simulink model "uc_faz_simetrik_PWM_simulink"  (R2019b)
settings: Solver=VariableStepAuto  StartTime=0.0  StopTime=0.02  RelTol=1e-3
values from neighbouring files (symbols this model uses):
  m = 0.70    (= 0.7)    [simetrikPWM_parametreleri.m]
  Ts = 1/2000    (= 0.0005)    [simetrikPWM_parametreleri.m]
  w = 2 * pi *50    (= 314.159265359)    [simetrikPWM_parametreleri.m]
libraries: powerlib x12
settings Model: Creator=Monster  LastModifiedBy=Monster

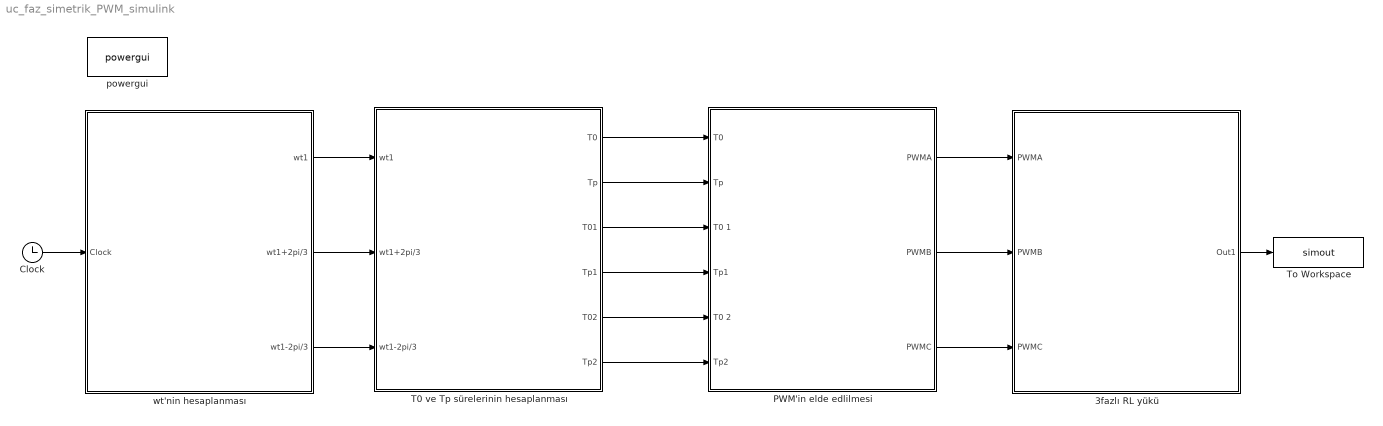
== system uc_faz_simetrik_PWM_simulink ==
  3fazlı RL yükü : Subsystem
  "Clock " : Clock
  PWM'in elde edlilmesi : Subsystem
  T0 ve Tp sürelerinin hesaplanması : Subsystem
  To Workspace : ToWorkspace  VariableName=simout  SaveFormat=Timeseries  SampleTime=-1
  "powergui " : powerlib/powergui  Priority=1  SimulationMode=Discrete  SampleTime=50e-6  frequency=60  Iterations=50  frequencyindice=0  Pbase=100e6  ErrMax=1e-4  UnitsV=kV  UnitsW=MW  buscounter=0  FunctionMessages=off  echomessages=off  EnableUseOfTLC=off  CurrentSourceSwitches=off  DisableSnubberDevices=off  DisableRonSwitches=off  DisableVfSwitches=off  DisplayEquations=off  AutomaticDiscreteSolvers=off  SolverType=Tustin/Backward Euler (TBE)  Interpol=off  ExternalGateDelay=off  methode=off  Ts=100  x0status=blocks  SPID=on  SwTol=0  HookPort=off  NonlinearTolerance=1e-4  nMaxIteration=100  ContinueOnMaxIteration=off  RestoreLinks=warning  ResistiveCurrentMeasurement=off  Frange=[0:2:500]  Ylog=off  Xlog=on  ShowGrid=off  save=off  variable=ZData  structure=0  ZoomFFT=off  StartTime=0.0  cycles=1  DisplayStyle=1  fundamental=60  FreqAxis=off  MaxFrequency=1000  frequencyindicesteady=1  RmsSteady=1  display=off
      settings: SourceProductName=Simscape Electrical
  wt'nin hesaplanması : Subsystem
  wires:
  "Clock "/1 -> wt'nin hesaplanması/1(Clock)
  wt'nin hesaplanması/1(wt1) -> T0 ve Tp sürelerinin hesaplanması/1(wt1)
  T0 ve Tp sürelerinin hesaplanması/1(T0) -> PWM'in elde edlilmesi/1("T0 ")
  T0 ve Tp sürelerinin hesaplanması/2(Tp) -> PWM'in elde edlilmesi/2(Tp)
  wt'nin hesaplanması/2(wt1+2pi/3) -> T0 ve Tp sürelerinin hesaplanması/2(wt1+2pi/3)
  wt'nin hesaplanması/3(wt1-2pi/3) -> T0 ve Tp sürelerinin hesaplanması/3(wt1-2pi/3)
  T0 ve Tp sürelerinin hesaplanması/3(T01) -> PWM'in elde edlilmesi/3(T0 1)
  T0 ve Tp sürelerinin hesaplanması/4(Tp1) -> PWM'in elde edlilmesi/4(Tp1)
  T0 ve Tp sürelerinin hesaplanması/5(T02) -> PWM'in elde edlilmesi/5(T0 2)
  T0 ve Tp sürelerinin hesaplanması/6(Tp2) -> PWM'in elde edlilmesi/6(Tp2)
  PWM'in elde edlilmesi/1(PWMA) -> 3fazlı RL yükü/1(PWMA)
  PWM'in elde edlilmesi/2(PWMB) -> 3fazlı RL yükü/2(PWMB)
  PWM'in elde edlilmesi/3(PWMC) -> 3fazlı RL yükü/3(PWMC)
  3fazlı RL yükü/1(Out1) -> To Workspace/1

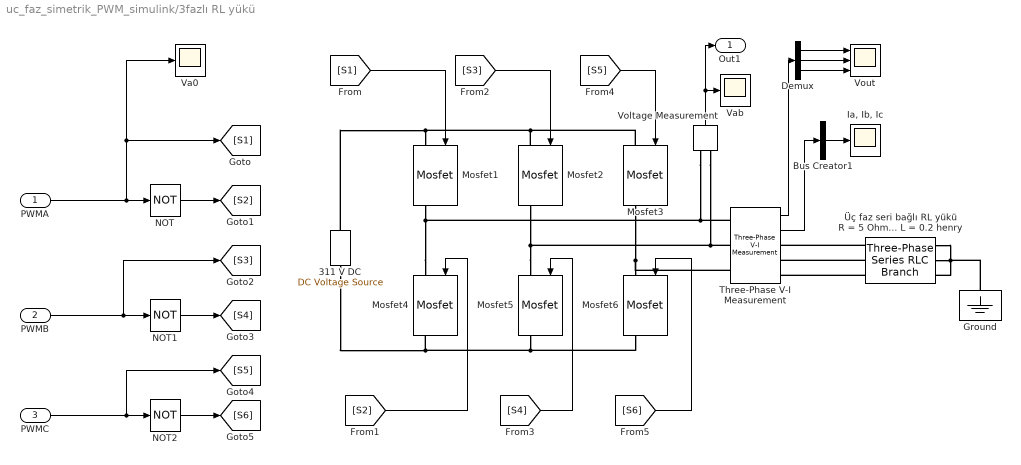
== system uc_faz_simetrik_PWM_simulink/3fazlı RL yükü ==
  PWMA : Inport
  PWMB : Inport  Port=2
  PWMC : Inport  Port=3
  311 V DC : powerlib/Electrical Sources/DC Voltage Source  Amplitude=311  Measurements=None
      settings: SourceProductName=Simscape Electrical
  Bus Creator1 : BusCreator  Inputs=1
  Demux : Demux  Outputs=3
  Ground : powerlib/Elements/Ground  LConnTagsString=a
      settings: SourceProductName=Simscape Electrical
  "Ia, Ib, Ic" : Scope
  "Mosfet1  " : powerlib/Power Electronics/Mosfet  Ron=0.1  Lon=0  Rd=0.01  Vfd=0  IC=0  Rs=1e5  Cs=inf  Measurements=on
      settings: SourceProductName=Simscape Electrical
  "Mosfet2  " : powerlib/Power Electronics/Mosfet  Ron=0.1  Lon=0  Rd=0.01  Vfd=0  IC=0  Rs=1e5  Cs=inf  Measurements=on
      settings: SourceProductName=Simscape Electrical
  "Mosfet3  " : powerlib/Power Electronics/Mosfet  Ron=0.1  Lon=0  Rd=0.01  Vfd=0  IC=0  Rs=1e5  Cs=inf  Measurements=on
      settings: SourceProductName=Simscape Electrical
  "Mosfet4  " : powerlib/Power Electronics/Mosfet  Ron=0.1  Lon=0  Rd=0.01  Vfd=0  IC=0  Rs=1e5  Cs=inf  Measurements=on
      settings: SourceProductName=Simscape Electrical
  "Mosfet5  " : powerlib/Power Electronics/Mosfet  Ron=0.1  Lon=0  Rd=0.01  Vfd=0  IC=0  Rs=1e5  Cs=inf  Measurements=on
      settings: SourceProductName=Simscape Electrical
  "Mosfet6  " : powerlib/Power Electronics/Mosfet  Ron=0.1  Lon=0  Rd=0.01  Vfd=0  IC=0  Rs=1e5  Cs=inf  Measurements=on
      settings: SourceProductName=Simscape Electrical
  NOT : Logic  Operator=NOT  AllPortsSameDT=off  OutDataTypeStr=boolean
  NOT1 : Logic  Operator=NOT  AllPortsSameDT=off  OutDataTypeStr=boolean
  NOT2 : Logic  Operator=NOT  AllPortsSameDT=off  OutDataTypeStr=boolean
  Three-Phase V-I Measurement : powerlib/Measurements/Three-Phase V-I Measurement  VoltageMeasurement=phase-to-ground  SetLabelV=off  LabelV=Vabc  Vpu=off  VpuLL=off  CurrentMeasurement=yes  SetLabelI=off  LabelI=Iabc  Ipu=off  Pbase=100e6  Vbase=500e3  OutputType=Complex  PhasorSimulation=off  PSBequivalent=0
      settings: SourceProductName=Simscape Electrical
  Va0 : Scope
  Vab : Scope
  Voltage Measurement : powerlib/Measurements/Voltage Measurement  PhasorSimulation=off  OutputType=Complex  PSBequivalent=0
      settings: SourceProductName=Simscape Electrical
  Vout : Scope  NumInputPorts=3
  Üç faz seri bağlı RL yükü R = 5 Ohm L = 0.2 henry : powerlib/Elements/Three-Phase Series RLC Branch  LConnTagsString=A|B|C  RConnTagsString=A|B|C  BranchType=RL  Resistance=5  Inductance=0.2  Capacitance=1e-6  Measurements=None
      settings: SourceProductName=Simscape Electrical
  Out1 : Outport
  wires:
  Voltage Measurement/1 -> Out1/1, Vab/1
  Demux/3 -> Vout/3
  [S3] -> "Mosfet2  "/1
  Three-Phase V-I Measurement/1 -> Demux/1
  [S6] -> "Mosfet6  "/1
  [S5] -> "Mosfet3  "/1
  Three-Phase V-I Measurement/2 -> Bus Creator1/1
  Demux/2 -> Vout/2
  Demux/1 -> Vout/1
  [S4] -> "Mosfet5  "/1
  [S2] -> "Mosfet4  "/1
  [S1] -> "Mosfet1  "/1
  Bus Creator1/1 -> "Ia, Ib, Ic"/1
  PWMA/1 -> [S1], Va0/1, NOT/1
  PWMB/1 -> [S3], NOT1/1
  PWMC/1 -> [S5], NOT2/1
  NOT/1 -> [S2]
  NOT1/1 -> [S4]
  NOT2/1 -> [S6]
  connections:
  "Mosfet2  "/LConn1 -- 311 V DC/RConn1 -- "Mosfet1  "/LConn1 -- "Mosfet3  "/LConn1
  "Mosfet4  "/LConn1 -- "Mosfet1  "/RConn1 -- Three-Phase V-I Measurement/LConn1 -- Voltage Measurement/LConn1
  Üç faz seri bağlı RL yükü R = 5 Ohm L = 0.2 henry/RConn3 -- Üç faz seri bağlı RL yükü R = 5 Ohm L = 0.2 henry/RConn1 -- Ground/LConn1 -- Üç faz seri bağlı RL yükü R = 5 Ohm L = 0.2 henry/RConn2
  "Mosfet6  "/LConn1 -- "Mosfet3  "/RConn1 -- Three-Phase V-I Measurement/LConn3
  "Mosfet4  "/RConn1 -- 311 V DC/LConn1 -- "Mosfet6  "/RConn1 -- "Mosfet5  "/RConn1
  "Mosfet5  "/LConn1 -- "Mosfet2  "/RConn1 -- Three-Phase V-I Measurement/LConn2 -- Voltage Measurement/LConn2
  Üç faz seri bağlı RL yükü R = 5 Ohm L = 0.2 henry/LConn1 -- Three-Phase V-I Measurement/RConn1
  Üç faz seri bağlı RL yükü R = 5 Ohm L = 0.2 henry/LConn2 -- Three-Phase V-I Measurement/RConn2
  Üç faz seri bağlı RL yükü R = 5 Ohm L = 0.2 henry/LConn3 -- Three-Phase V-I Measurement/RConn3

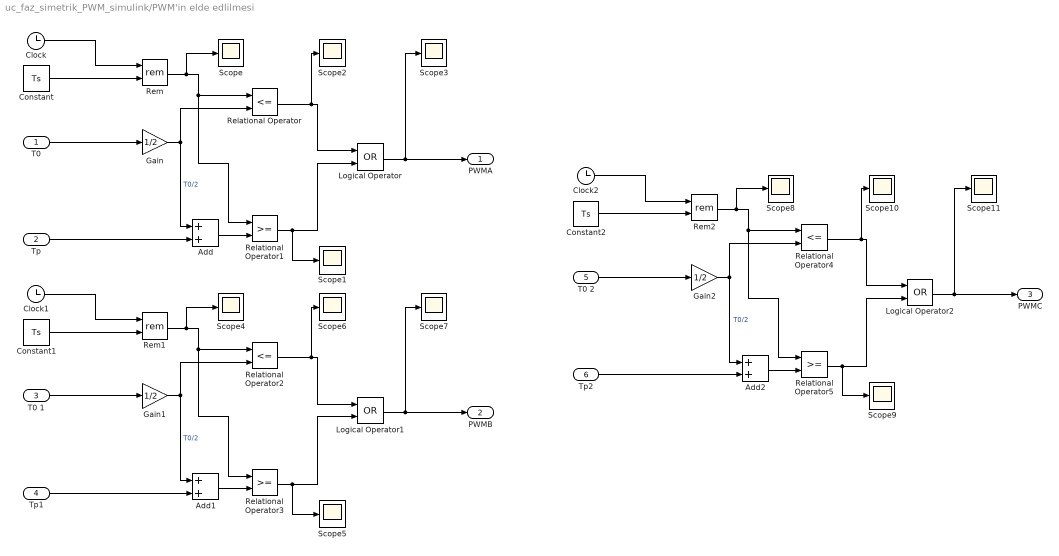
== system uc_faz_simetrik_PWM_simulink/PWM'in elde edlilmesi ==
  "T0 " : Inport
  Tp : Inport  Port=2
  T0 1 : Inport  Port=3
  Tp1 : Inport  Port=4
  T0 2 : Inport  Port=5
  Tp2 : Inport  Port=6
  Add : Sum
  Add1 : Sum
  Add2 : Sum
  Clock : Clock
  Clock1 : Clock
  Clock2 : Clock
  Constant : Constant  Value=Ts
  Constant1 : Constant  Value=Ts
  Constant2 : Constant  Value=Ts
  Gain : Gain  Gain=1/2
  Gain1 : Gain  Gain=1/2
  Gain2 : Gain  Gain=1/2
  Logical Operator : Logic  Operator=OR  AllPortsSameDT=off  OutDataTypeStr=boolean
  Logical Operator1 : Logic  Operator=OR  AllPortsSameDT=off  OutDataTypeStr=boolean
  Logical Operator2 : Logic  Operator=OR  AllPortsSameDT=off  OutDataTypeStr=boolean
  "Relational Operator " : RelationalOperator  Operator=<=  OutDataTypeStr=boolean  RndMeth=Simplest
  Relational Operator1 : RelationalOperator  OutDataTypeStr=boolean  RndMeth=Simplest
  Relational Operator2 : RelationalOperator  Operator=<=  OutDataTypeStr=boolean  RndMeth=Simplest
  Relational Operator3 : RelationalOperator  OutDataTypeStr=boolean  RndMeth=Simplest
  Relational Operator4 : RelationalOperator  Operator=<=  OutDataTypeStr=boolean  RndMeth=Simplest
  Relational Operator5 : RelationalOperator  OutDataTypeStr=boolean  RndMeth=Simplest
  "Rem " : Math  Operator=rem  SignedPower=off  SaturateOnIntegerOverflow=on
  Rem1 : Math  Operator=rem  SignedPower=off  SaturateOnIntegerOverflow=on
  Rem2 : Math  Operator=rem  SignedPower=off  SaturateOnIntegerOverflow=on
  Scope{,1..11} (12 alike) : Scope
  PWMA : Outport
  PWMB : Outport  Port=2
  PWMC : Outport  Port=3
  wires:
  "T0 "/1 -> Gain/1
  Constant/1 -> "Rem "/2
  Clock/1 -> "Rem "/1
  "Rem "/1 -> Scope/1, "Relational Operator "/1, Relational Operator1/1
  Gain/1 -> Add/1, "Relational Operator "/2  "T0/2"
  Logical Operator/1 -> PWMA/1, Scope3/1
  Tp/1 -> Add/2
  Add/1 -> Relational Operator1/2
  Relational Operator1/1 -> Scope1/1, Logical Operator/2
  "Relational Operator "/1 -> Scope2/1, Logical Operator/1
  Relational Operator2/1 -> Logical Operator1/1, Scope6/1
  Relational Operator3/1 -> Logical Operator1/2, Scope5/1
  Add1/1 -> Relational Operator3/2
  Tp1/1 -> Add1/2
  Logical Operator1/1 -> Scope7/1, PWMB/1
  Gain1/1 -> Relational Operator2/2, Add1/1  "T0/2"
  Rem1/1 -> Relational Operator3/1, Relational Operator2/1, Scope4/1
  Clock1/1 -> Rem1/1
  Constant1/1 -> Rem1/2
  T0 1/1 -> Gain1/1
  T0 2/1 -> Gain2/1
  Constant2/1 -> Rem2/2
  Clock2/1 -> Rem2/1
  Rem2/1 -> Scope8/1, Relational Operator4/1, Relational Operator5/1
  Gain2/1 -> Add2/1, Relational Operator4/2  "T0/2"
  Logical Operator2/1 -> PWMC/1, Scope11/1
  Tp2/1 -> Add2/2
  Add2/1 -> Relational Operator5/2
  Relational Operator5/1 -> Scope9/1, Logical Operator2/2
  Relational Operator4/1 -> Scope10/1, Logical Operator2/1

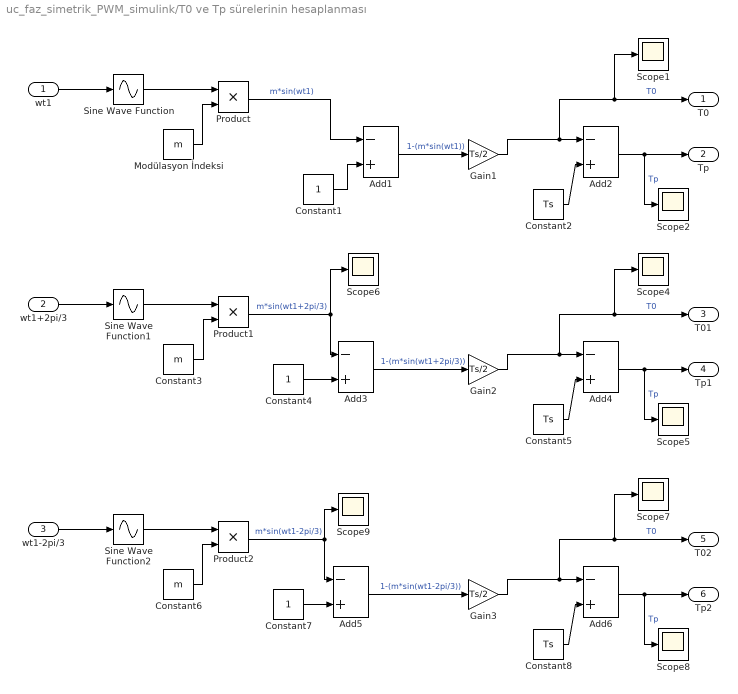
== system uc_faz_simetrik_PWM_simulink/T0 ve Tp sürelerinin hesaplanması ==
  wt1 : Inport
  wt1+2pi/3 : Inport  Port=2
  wt1-2pi/3 : Inport  Port=3
  Add{1..6} (6 alike) : Sum  Inputs=-+
  Constant1 : Constant
  Constant2 : Constant  Value=Ts
  Constant3 : Constant  Value=m
  Constant4 : Constant
  Constant5 : Constant  Value=Ts
  Constant6 : Constant  Value=m
  Constant7 : Constant
  Constant8 : Constant  Value=Ts
  Gain1 : Gain  Gain=Ts/2
  Gain2 : Gain  Gain=Ts/2
  Gain3 : Gain  Gain=Ts/2
  Modülasyon İndeksi : Constant  Value=m
  Product : Product
  Product1 : Product
  Product2 : Product
  Scope{1..2,4..9} (8 alike) : Scope
  "Sine Wave Function " : Sin  TimeSource=Use external signal  SampleTime=0
  Sine Wave Function1 : Sin  TimeSource=Use external signal  SampleTime=0
  Sine Wave Function2 : Sin  TimeSource=Use external signal  SampleTime=0
  T0 : Outport
  Tp : Outport  Port=2
  T01 : Outport  Port=3
  Tp1 : Outport  Port=4
  T02 : Outport  Port=5
  Tp2 : Outport  Port=6
  wires:
  wt1/1 -> "Sine Wave Function "/1
  Add1/1 -> Gain1/1  "1-(m*sin(wt1))"
  Constant1/1 -> Add1/2
  Gain1/1 -> T0/1, Scope1/1, Add2/1  "T0"
  Constant2/1 -> Add2/2
  Add2/1 -> Tp/1, Scope2/1  "Tp"
  "Sine Wave Function "/1 -> Product/1
  Modülasyon İndeksi/1 -> Product/2
  Product/1 -> Add1/1  "m*sin(wt1)"
  Product1/1 -> Add3/1, Scope6/1  "m*sin(wt1+2pi/3)"
  Constant3/1 -> Product1/2
  Sine Wave Function1/1 -> Product1/1
  Add4/1 -> Scope5/1, Tp1/1  "Tp"
  Constant5/1 -> Add4/2
  Gain2/1 -> Add4/1, Scope4/1, T01/1  "T0"
  Constant4/1 -> Add3/2
  Add3/1 -> Gain2/1  "1-(m*sin(wt1+2pi/3))"
  wt1+2pi/3/1 -> Sine Wave Function1/1
  wt1-2pi/3/1 -> Sine Wave Function2/1
  Add5/1 -> Gain3/1  "1-(m*sin(wt1-2pi/3))"
  Constant7/1 -> Add5/2
  Gain3/1 -> T02/1, Scope7/1, Add6/1  "T0"
  Constant8/1 -> Add6/2
  Add6/1 -> Tp2/1, Scope8/1  "Tp"
  Sine Wave Function2/1 -> Product2/1
  Constant6/1 -> Product2/2
  Product2/1 -> Scope9/1, Add5/1  "m*sin(wt1-2pi/3)"

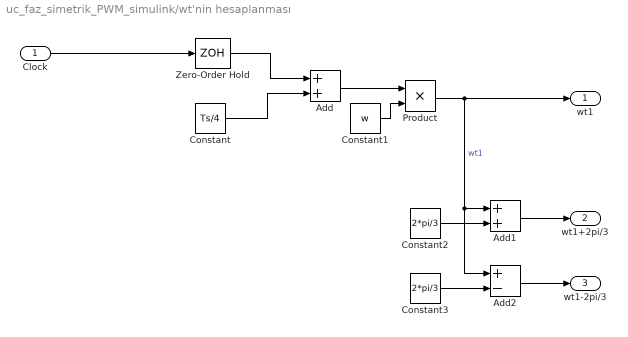
== system uc_faz_simetrik_PWM_simulink/wt'nin hesaplanması ==
  Clock : Inport
  "Add " : Sum
  Add1 : Sum
  Add2 : Sum  Inputs=+-
  "Constant " : Constant  Value=Ts/4
  Constant1 : Constant  Value=w
  Constant2 : Constant  Value=2*pi/3
  Constant3 : Constant  Value=2*pi/3
  Product : Product
  "Zero-Order Hold " : ZeroOrderHold  SampleTime=Ts
  wt1 : Outport
  wt1+2pi/3 : Outport  Port=2
  wt1-2pi/3 : Outport  Port=3
  wires:
  Clock/1 -> "Zero-Order Hold "/1
  "Zero-Order Hold "/1 -> "Add "/1
  "Constant "/1 -> "Add "/2
  "Add "/1 -> Product/1
  Constant1/1 -> Product/2
  Constant2/1 -> Add1/2
  Add1/1 -> wt1+2pi/3/1
  Constant3/1 -> Add2/2
  Product/1 -> Add2/1, Add1/1, wt1/1  "wt1"
  Add2/1 -> wt1-2pi/3/1
